simulink model "Encoder_RPM"  (R2024b)
settings: Solver=FixedStepAuto  StartTime=0.0  StopTime=inf  FixedStep=0.0001  MaxStep=0.005  RelTol=1e-3  EnableMultiTasking=on
libraries: simulink x1, arduinolib x1
settings Model: ExtModeBatchMode=on  ExtModeTrigDuration=2  Creator=jesus  LastModifiedBy=jesus
settings SolverCC: AutoInsertRateTranBlk=on
settings OptimizationCC: EnhancedBackFolding=on  PassReuseOutputArgsAs=Individual arguments  ZeroExternalMemoryAtStartup=off  ZeroInternalMemoryAtStartup=off  MaxStackSize=64  OptimizeBlockOrder=speed  DifferentSizesBufferReuse=on  OptimizationCustomize=off  EfficientTunableParamExpr=on
settings DebuggingCC: ParameterTunabilityLossMsg=error
settings HardwareCC: ProdBitPerInt=16  ProdBitPerPointer=16  ProdBitPerSizeT=16  ProdBitPerPtrDiffT=16  ProdLargestAtomicFloat=None  ProdWordSize=8  ProdHWDeviceType=Atmel->AVR
settings SFSimCC: MATLABDynamicMemAlloc=off
settings RTWCC: Description=Embedded Coder  SystemTargetFile=ert.tlc  HardwareBoard=Arduino Mega 2560  TemplateMakefile=ert_default_tmf  Toolchain=Arduino AVR  BuildConfiguration=Faster Runs
settings CodeAppCC: ForceParamTrailComments=on  IgnoreCustomStorageClasses=off  OperatorAnnotations=on  SimulinkDataObjDesc=on  SFDataObjDesc=on  InsertBlockDesc=on
settings ERTTargetCC: SupportContinuousTime=on  SupportVariableSizeSignals=on  ExtModeTransport=3  ExtModeStaticAlloc=on  ExtModeAutomaticAllocSize=off  ExtModeStaticAllocSize=2048  ExtModeMexFile=ext_xcp  ExtModeIntrfLevel=Level2 - Open  InlinedParameterPlacement=Hierarchical

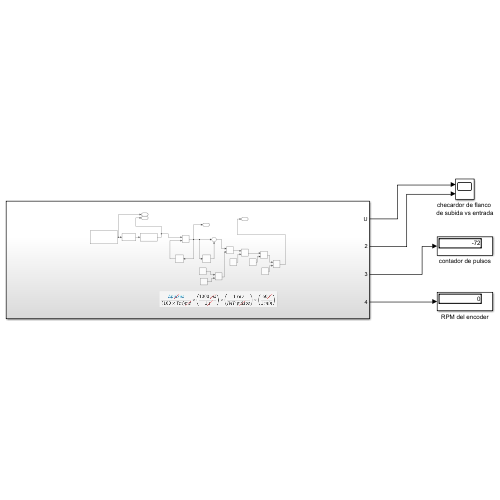
[thumbnail: Simulink's stored preview of the top-level diagram]
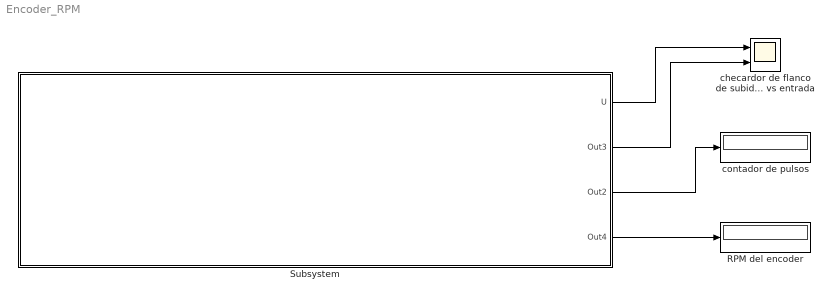
== system Encoder_RPM ==
  RPM del encoder : Display
  Subsystem : Subsystem
  checardor de flanco de subida vs entrada : Scope  NumInputPorts=2
  contador de pulsos : Display
  wires:
  Subsystem/1(U) -> checardor de flanco de subida vs entrada/1
  Subsystem/3(Out2) -> contador de pulsos/1
  Subsystem/2(Out3) -> checardor de flanco de subida vs entrada/2
  Subsystem/4(Out4) -> RPM del encoder/1

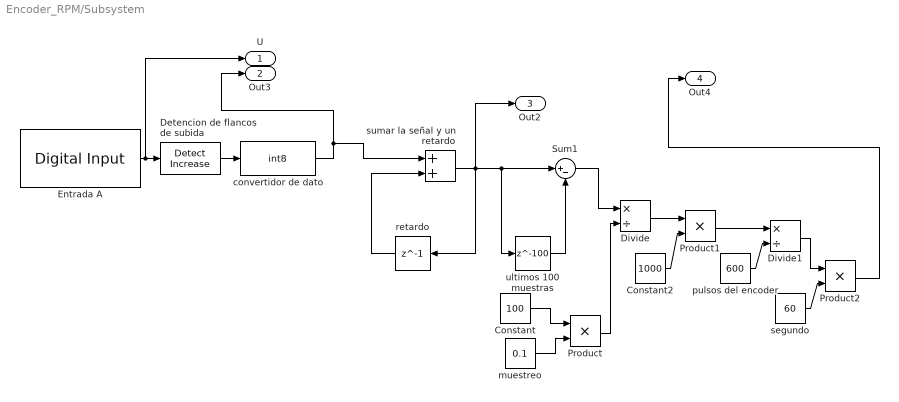
== system Encoder_RPM/Subsystem ==
  Constant : Constant  Value=100
  Constant2 : Constant  Value=1000
  Detencion de flancos de subida : simulink/Logic and Bit Operations/Detect Increase  vinit=0.0  OutDataTypeStr=boolean
  Divide : Product  Inputs=*/
  Divide1 : Product  Inputs=*/
  Entrada A : arduinolib/Digital Input  pinNumber=7  mode=Input Pullup  Direction=input  SampleTime=0.0001  blockPlatform=arduino
  Product : Product
  Product1 : Product
  Product2 : Product
  Sum1 : Sum  Inputs=|+-
  convertidor de dato : DataTypeConversion  OutDataTypeStr=int8  SaturateOnIntegerOverflow=off  RndMeth=Floor
  muestreo : Constant  Value=0.1
  pulsos del encoder : Constant  Value=600
  retardo : Delay  DelayLength=1
  segundo : Constant  Value=60
  sumar la señal y un retardo : Sum
  ultimos 100 muestras : Delay  DelayLength=100
  U : Outport
  Out3 : Outport  Port=2
  Out2 : Outport  Port=3
  Out4 : Outport  Port=4
  wires:
  Detencion de flancos de subida/1 -> convertidor de dato/1
  sumar la señal y un retardo/1 -> Out2/1, ultimos 100 muestras/1, Sum1/1, retardo/1
  Product/1 -> Divide/2
  convertidor de dato/1 -> Out3/1, sumar la señal y un retardo/1
  Entrada A/1 -> U/1, Detencion de flancos de subida/1
  Constant/1 -> Product/1
  ultimos 100 muestras/1 -> Sum1/2
  retardo/1 -> sumar la señal y un retardo/2
  segundo/1 -> Product2/2
  muestreo/1 -> Product/2
  Sum1/1 -> Divide/1
  Product1/1 -> Divide1/1
  Divide1/1 -> Product2/1
  Divide/1 -> Product1/1
  Constant2/1 -> Product1/2
  pulsos del encoder/1 -> Divide1/2
  Product2/1 -> Out4/1
